simulink library "Storage_Type_4"  (R2016b)
settings: Solver=ode45  StartTime=0.0  StopTime=10.0  RelTol=1e-3  EnableMultiTasking=on
libraries: carnot x9
settings Model: Creator=lena.frank  LastModifiedBy=drhf
settings DataIOCC: LimitDataPoints=on  SaveFormat=Array  SignalLoggingSaveFormat=ModelDataLogs
settings OptimizationCC: ExpressionDepthLimit=2147483647  LifeSpan=inf
settings DebuggingCC: UnderspecifiedInitializationDetection=Classic  MergeDetectMultiDrivingBlocksExec=none  SolverPrmCheckMsg=warning  FcnCallInpInsideContextMsg=warning  StateNameClashWarn=warning  SFUnexpectedBacktrackingDiag=warning  SFNoUnconditionalDefaultTransitionDiag=warning  SFExecutionAtInitializationDiag=none
settings HardwareCC: ProdBitPerPointer=32  ProdBitPerSizeT=32  ProdBitPerPtrDiffT=32  ProdLargestAtomicFloat=None  ProdIntDivRoundTo=Undefined  ProdEndianess=Unspecified  ProdWordSize=32  ProdHWDeviceType=32-bit Generic
settings ModelReferenceCC: PropagateSignalLabelsOutOfModel=off
settings GRTTargetCC: TargetLangStandard=C89/C90 (ANSI)  GeneratePreprocessorConditionals=Disable all  CombineOutputUpdateFcns=off  GRTInterface=on
settings ConfigComp: CovMetricSettings=dw  CovHtmlReporting=on  CovSaveCumulativeToWorkspaceVar=on  CovSaveSingleToWorkspaceVar=on  CovExternalEMLEnable=off

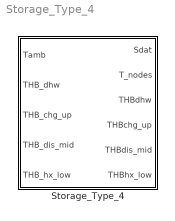
== system Storage_Type_4 ==
  Storage_Type_4 : Subsystem  mask(Multiport Storage){uloss=1, ubot=1, utop=1, cond=1, volume=0.5, dia=0.5, pos=standing cylinder, h_in1=1, h_out1=0.54, dia1pipe=0.04, h_in2=0.45, h_out2=0, ua0_2=678.6, uam_2=0.411, uat_2=0.287, dplin_2=100, dpqua_2=100, h_in3=0.45, h_out3=0.54, dia3pipe=0.04, h_in4=0.02, h_out4=0.95, ua0_4=642.2, uam_4=0.369, uat_4=0.684, dplin4=100, dpqua=100, t0=[10:5:55], nodes=50, mpoints=50}
      mask prompts: uloss "Heat transfer coefficient to ambient [W/m²K]"; ubot "Heat transfer coefficient to ambient bottom [W/m²K]"; utop "Heat transfer coefficient to ambient top [W/m²K]"; cond "Effective thermal conductivity [W/m/K]"; volume "Volume [m³]"; dia "Diameter [m]"; pos "Position"; h_in1 "relative height of inlet, range from 0 (= bottom) to 1 (= top)"; h_out1 "relative height of outlet, range from 0 (= bottom) to 1 (= top)"; dia1pipe "Diameter of pipe in m"; h_in2 "relative height of inlet, range from 0 (= bottom) to 1 (= top)"; h_out2 "relative height of outlet, range from 0 (= bottom) to 1 (= top)"; ua0_2 "uac: heat transfer coefficient [W/K /(kg/s) /(°C)]"; uam_2 "uam: massflow dependent heat transfer [-]"; uat_2 "uat: temperature difference dependent heat transfer [-]"; dplin_2 "pressure drop linear in mdot [Pa*s/kg]"; dpqua_2 "pressure drop quadratic in mdot [Pa*s²/kg²]"; h_in3 "relative height of inlet, range from 0 (= bottom) to 1 (= top)"; h_out3 "relative height of outlet, range from 0 (= bottom) to 1 (= top)"; dia3pipe "Diameter of pipe in m"; h_in4 "relative height of inlet, range from 0 (= bottom) to 1 (= top)"; h_out4 "relative height of outlet, range from 0 (= bottom) to 1 (= top)"; ua0_4 "uac: heat transfer coefficient [W/K /(kg/s) /(°C)]"; uam_4 "uam: massflow dependent heat transfer [-]"; uat_4 "uat: temperature difference dependent heat transfer [-]"; dplin4 "pressure drop linear in mdot [Pa*s/kg]"; dpqua "pressure drop quadratic in mdot [Pa*s²/kg²]"; t0 "Initial temperature (vector or scalar) in °C"; nodes "number of nodes"; mpoints "Number of measurement points"
      mask help:
      | The volmue of the cylindrical storage is divided in a number "nodes" of horizontal slices (1xN-node model). For each node the energy balance equation is solved.
      | Parameters from underlying sub-masks are promoted by top mask.
      mask init:
      | [standing, dh, height, mpts, tini] ...
      |     = CarnotCallbacks_StorageTypeN(pos, volume, dia, nodes, mpoints, t0);
      mask Help: web(fullfile(path_carnot('help'),'Storage_Type_N.html'),'-helpbrowser')
      mask TypeOptions uloss: sfun_storageTnodes/uloss
      mask TypeOptions ubot: sfun_storageTnodes/ubot
      mask TypeOptions utop: sfun_storageTnodes/utop
      mask TypeOptions cond: sfun_storageTnodes/cond
      mask TypeOptions volume: sfun_storageTnodes/volume | CreateSdat/volume
      mask TypeOptions dia: sfun_storageTnodes/dia
      mask TypeOptions pos: lying cylinder | standing cylinder
      mask TypeOptions h_in1: pipe_charge_up/h_in
      mask TypeOptions h_out1: pipe_charge_up/h_out
      mask TypeOptions dia1pipe: pipe_charge_up/dia
      mask TypeOptions h_in2: HX_EN12977_solar/h_in
      mask TypeOptions h_out2: HX_EN12977_solar/h_out
      mask TypeOptions ua0_2: HX_EN12977_solar/ua0
      mask TypeOptions uam_2: HX_EN12977_solar/uam
      mask TypeOptions uat_2: HX_EN12977_solar/uat
      mask TypeOptions dplin_2: HX_EN12977_solar/dplin
      mask TypeOptions dpqua_2: HX_EN12977_solar/dpqua
      mask TypeOptions h_in3: pipe_heating/h_in
      mask TypeOptions h_out3: pipe_heating/h_out
      mask TypeOptions dia3pipe: pipe_heating/dia
      mask TypeOptions h_in4: HX_EN12977_dhw/h_in
      mask TypeOptions h_out4: HX_EN12977_dhw/h_out
      mask TypeOptions ua0_4: HX_EN12977_dhw/ua0
      mask TypeOptions uam_4: HX_EN12977_dhw/uam
      mask TypeOptions uat_4: HX_EN12977_dhw/uat
      mask TypeOptions dplin4: HX_EN12977_dhw/dplin
      mask TypeOptions dpqua: HX_EN12977_dhw/dpqua
      mask TypeOptions nodes: sfun_storageTnodes/nodes
      mask Display: plot(5,10,85,110,[36,36,40,50,54,54,50,40,36],[90,50,45,45,50,90,93,93,90],[36,51,40,51,36],[50,50,68,85,85],[36,51,44,51,36],[54,54,56,58,58])

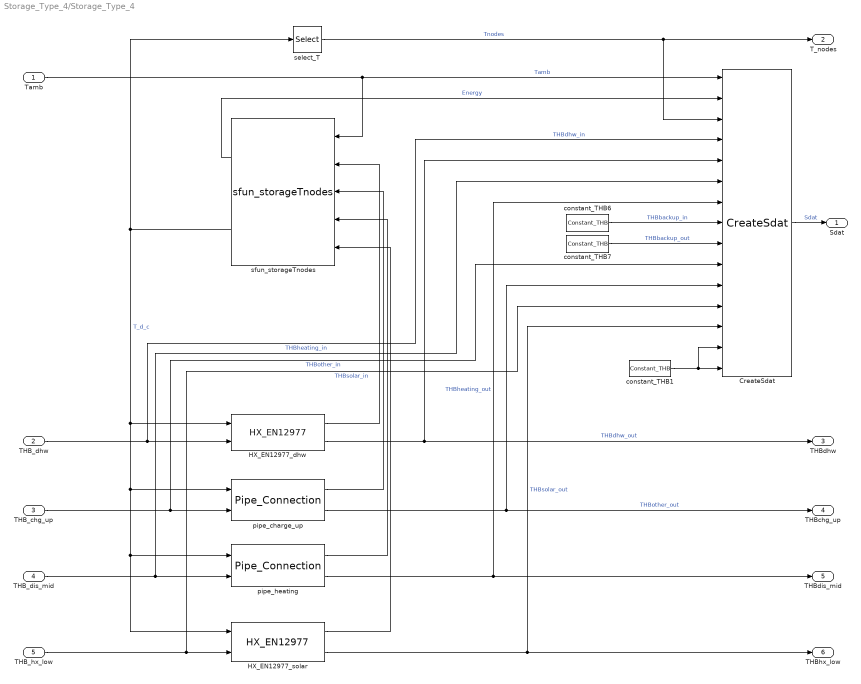
== system Storage_Type_4/Storage_Type_4 ==
  Tamb : Inport
  THB_dhw : Inport  Port=2
  THB_chg_up : Inport  Port=3
  THB_dis_mid : Inport  Port=4
  THB_hx_low : Inport  Port=5
  CreateSdat : carnot/Basic/Thermal_Models/CreateSdat  volume=volume  stgtype=1
  HX_EN12977_dhw : carnot/Storage/Thermal/Storage_Ports/HX_EN12977  h_in=h_in4  h_out=h_out4  hgt=height  dia=dia  ua0=ua0_4  uam=uam_4  uat=uat_4  dplin=dplin4  dpqua=dpqua  nodes=nodes
  HX_EN12977_solar : carnot/Storage/Thermal/Storage_Ports/HX_EN12977  h_in=h_in2  h_out=h_out2  hgt=height  dia=dia  ua0=ua0_2  uam=uam_2  uat=uat_2  dplin=dplin_2  dpqua=dpqua_2  nodes=nodes
  constant_THB1 : carnot/Source/Simple/Constant_THB  t=20  mdot=0  p=1e5  mID=No Pressure Drop  fluid=Water  mix=0  mix2=0  mix3=0  dia=0.02  hgt=0
  constant_THB6 : carnot/Source/Simple/Constant_THB  t=20  mdot=0  p=1e5  mID=No Pressure Drop  fluid=Water  mix=0  mix2=0  mix3=0  dia=0.02  hgt=0
  constant_THB7 : carnot/Source/Simple/Constant_THB  t=20  mdot=0  p=1e5  mID=No Pressure Drop  fluid=Water  mix=0  mix2=0  mix3=0  dia=0.02  hgt=0
  pipe_charge_up : carnot/Storage/Thermal/Storage_Ports/Pipe_Connection  h_in=h_in1  h_out=h_out1  hgt=height  dia=dia1pipe  nodes=nodes
  pipe_heating : carnot/Storage/Thermal/Storage_Ports/Pipe_Connection  h_in=h_in3  h_out=h_out3  hgt=height  dia=dia3pipe  nodes=nodes
  select_T : Selector  InputPortWidth=nodes  IndexOptions=Index vector (dialog)  Indices=mpts  OutputSizes=1
  sfun_storageTnodes : carnot/Basic/Thermal_Models/sfun_storageTnodes  uloss=uloss  ubot=ubot  utop=utop  cond=cond  volume=volume  dia=dia  standing=standing cylinder  tini=tini  nodes=nodes  nconnect=4  elimthermocline=2  condinvtc=1e5
  Sdat : Outport
  T_nodes : Outport  Port=2
  THBdhw : Outport  Port=3
  THBchg_up : Outport  Port=4
  THBdis_mid : Outport  Port=5
  THBhx_low : Outport  Port=6
  wires:
  constant_THB1/1 -> CreateSdat/15, CreateSdat/14
  constant_THB7/1 -> CreateSdat/9  "THBbackup_out"
  constant_THB6/1 -> CreateSdat/8  "THBbackup_in"
  pipe_heating/2 -> THBdis_mid/1, CreateSdat/7  "THBheating_out"
  HX_EN12977_solar/1 -> sfun_storageTnodes/5
  pipe_heating/1 -> sfun_storageTnodes/4
  THB_dis_mid/1 -> pipe_heating/2, CreateSdat/6  "THBheating_in"
  Tamb/1 -> CreateSdat/1, sfun_storageTnodes/1  "Tamb"
  THB_dhw/1 -> HX_EN12977_dhw/2, CreateSdat/4  "THBdhw_in"
  HX_EN12977_dhw/2 -> THBdhw/1, CreateSdat/5  "THBdhw_out"
  HX_EN12977_dhw/1 -> sfun_storageTnodes/2
  select_T/1 -> T_nodes/1, CreateSdat/3  "Tnodes"
  sfun_storageTnodes/1 -> CreateSdat/2  "Energy"
  sfun_storageTnodes/2 -> select_T/1, HX_EN12977_dhw/1, pipe_heating/1, HX_EN12977_solar/1, pipe_charge_up/1  "T_d_c"
  CreateSdat/1 -> Sdat/1  "Sdat"
  THB_chg_up/1 -> pipe_charge_up/2, CreateSdat/10  "THBother_in"
  pipe_charge_up/2 -> THBchg_up/1, CreateSdat/11  "THBother_out"
  pipe_charge_up/1 -> sfun_storageTnodes/3
  THB_hx_low/1 -> HX_EN12977_solar/2, CreateSdat/12  "THBsolar_in"
  HX_EN12977_solar/2 -> THBhx_low/1, CreateSdat/13  "THBsolar_out"
